simulink model "PC1_DynamicModel"  (R2024b)
settings: Solver=ode45  StartTime=0.0  StopTime=1000  RelTol=1e-3
settings Model: Creator=dereckbouchard  LastModifiedBy=dereckbouchard

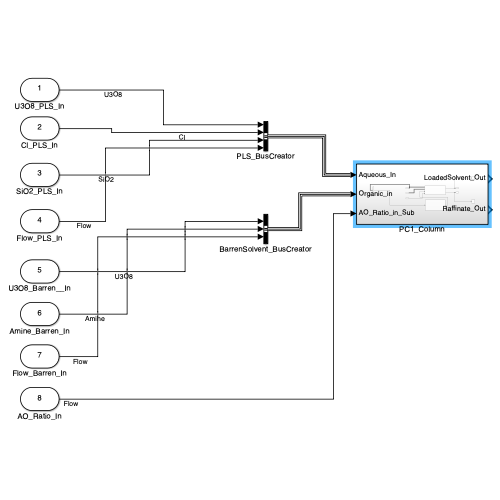
[thumbnail: Simulink's stored preview of the top-level diagram]
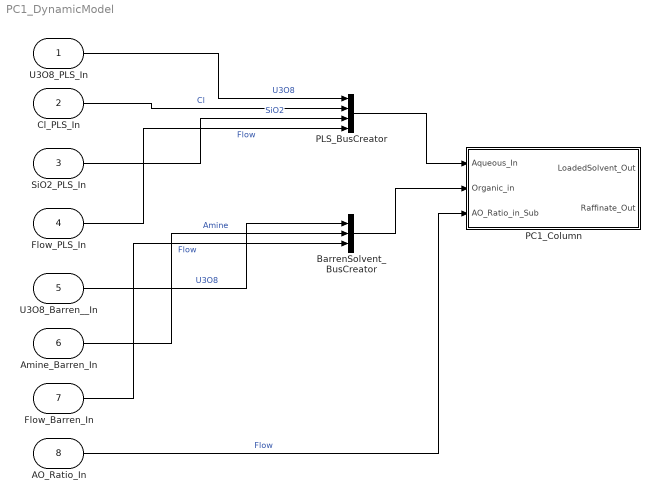
== system PC1_DynamicModel ==
  U3O8_PLS_In : Inport  OutDataTypeStr=double  PortDimensions=[1 1]  SampleTime=0
  Cl_PLS_In : Inport  Port=2  OutDataTypeStr=double  PortDimensions=[1 1]  SampleTime=0
  SiO2_PLS_In : Inport  Port=3  OutDataTypeStr=double  PortDimensions=[1 1]  SampleTime=0
  Flow_PLS_In : Inport  Port=4  OutDataTypeStr=double  PortDimensions=[1 1]  SampleTime=0
  U3O8_Barren__In : Inport  Port=5  OutDataTypeStr=double  PortDimensions=[1 1]  SampleTime=0
  Amine_Barren_In : Inport  Port=6  OutDataTypeStr=double  PortDimensions=[1 1]  SampleTime=0
  Flow_Barren_In : Inport  Port=7  OutDataTypeStr=double  PortDimensions=[1 1]  SampleTime=0
  AO_Ratio_In : Inport  Port=8  OutDataTypeStr=double  PortDimensions=[1 1]  SampleTime=0
  BarrenSolvent_BusCreator : BusCreator  Inputs=3  OutDataTypeStr=Bus: BarrenSolvent_Bus
  PC1_Column : Subsystem
  PLS_BusCreator : BusCreator  Inputs=4  OutDataTypeStr=Bus: PLS_Bus
      settings: InheritFromInputs=off
  wires:
  U3O8_PLS_In/1 -> PLS_BusCreator/1  "U3O8"
  Cl_PLS_In/1 -> PLS_BusCreator/2  "Cl"
  SiO2_PLS_In/1 -> PLS_BusCreator/3  "SiO2"
  Flow_PLS_In/1 -> PLS_BusCreator/4  "Flow"
  U3O8_Barren__In/1 -> BarrenSolvent_BusCreator/1  "U3O8"
  Amine_Barren_In/1 -> BarrenSolvent_BusCreator/2  "Amine"
  Flow_Barren_In/1 -> BarrenSolvent_BusCreator/3  "Flow"
  PLS_BusCreator/1 -> PC1_Column/1(Aqueous_In)
  BarrenSolvent_BusCreator/1 -> PC1_Column/2(Organic_in)
  AO_Ratio_In/1 -> PC1_Column/3(AO_Ratio_in_Sub)  "Flow"

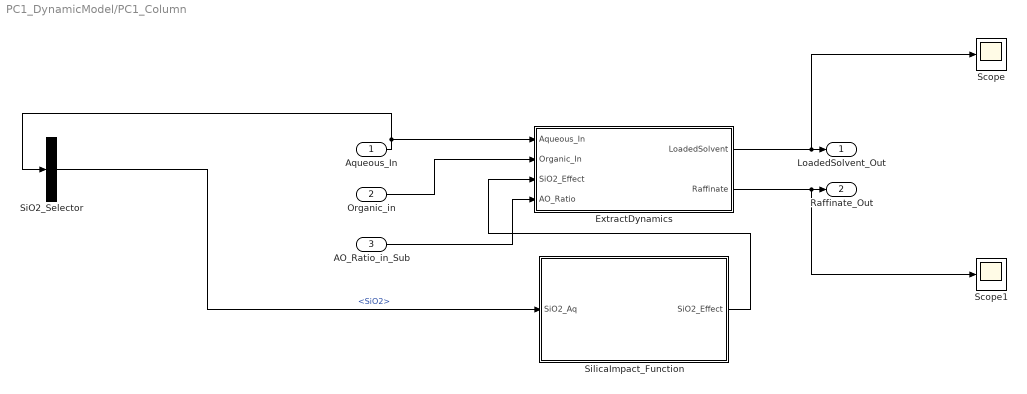
== system PC1_DynamicModel/PC1_Column ==
  Aqueous_In : Inport
  Organic_in : Inport  Port=2
  AO_Ratio_in_Sub : Inport  Port=3
  ExtractDynamics : MATLAB Function  TreatAsAtomicUnit=on
  Scope : Scope
  Scope1 : Scope
  SiO2_Selector : BusSelector  OutputSignals=SiO2
  SilicaImpact_Function : MATLAB Function  TreatAsAtomicUnit=on
  LoadedSolvent_Out : Outport  OutDataTypeStr=double  PortDimensions=[1 3]  SampleTime=0
  Raffinate_Out : Outport  Port=2  OutDataTypeStr=double  PortDimensions=[1 4]  SampleTime=0
  wires:
  Aqueous_In/1 -> SiO2_Selector/1, ExtractDynamics/1(Aqueous_In)
  Organic_in/1 -> ExtractDynamics/2(Organic_In)
  ExtractDynamics/1(LoadedSolvent) -> Scope/1, LoadedSolvent_Out/1
  ExtractDynamics/2(Raffinate) -> Scope1/1, Raffinate_Out/1
  SiO2_Selector/1 -> SilicaImpact_Function/1(SiO2_Aq)  "<SiO2>"
  SilicaImpact_Function/1(SiO2_Effect) -> ExtractDynamics/3(SiO2_Effect)
  AO_Ratio_in_Sub/1 -> ExtractDynamics/4(AO_Ratio)

== matlab function PC1_DynamicModel/PC1_Column/SilicaImpact_Function ==
  data: SiO2_Aq input; SiO2_Effect output
function SiO2_Effect = SilicaImpact(SiO2_Aq)
    % Simplified: Reduces extraction efficiency if SiO2 > 0.4 g/L
    if SiO2_Aq > 0.4
        SiO2_Effect = 0.9; % 10% reduction in efficiency (e.g., entrainment)
    else
        SiO2_Effect = 1.0; % No effect
    end
end

== matlab function PC1_DynamicModel/PC1_Column/ExtractDynamics ==
  data: Aqueous_In input; LoadedSolvent output; Organic_In input; Raffinate output; SiO2_Effect input; AO_Ratio input
function [LoadedSolvent, Raffinate] = ExtractDynamics(Aqueous_In, Organic_In, SiO2_Effect, AO_Ratio)
    % Inputs: Aqueous_In (bus with U3O8, Cl, SiO2, Flow), Organic_In (bus with U3O8, Amine, Flow), SiO2_Effect, AO_Ratio
    % Constants from plant data
    Amine_Conc = 0.06; % 6% amine concentration
    
    % Extract concentrations and flows from buses
    U3O8_Aq = Aqueous_In.U3O8; % mg/L
    Cl_Aq = Aqueous_In.Cl; % mg/L
    SiO2_Aq = Aqueous_In.SiO2; % g/L
    Flow_Aq = Aqueous_In.Flow; % m³/h
    U3O8_Org = Organic_In.U3O8; % mg/L
    Amine_Frac = Organic_In.Amine; % fraction (0.06)
    Flow_Org = Organic_In.Flow; % m³/h
    
    % Uranium extraction reaction (simplified), adjusted for silica and A/O ratio
    % [(R3NH+)_2SO4^2-] + UO2(SO4)2^2- -> [(R3NH+)_2UO2(SO4)2] + SO4^2-
    Max_U3O8_Org = 2500; % Target loaded solvent U3O8 (midpoint of 2100–3150 mg/L)
    U3O8_Extracted = min(U3O8_Aq * (Flow_Aq / (Flow_Aq + Flow_Org * AO_Ratio)), Amine_Frac * 1000 * 1000) * SiO2_Effect;
    
    % Chloride competition reaction
    % [(R3NH+)_2SO4^2-] + Cl- -> (R3NH+Cl-) + SO4^2-
    Cl_Competed = min(Cl_Aq * (Flow_Aq / (Flow_Aq + Flow_Org * AO_Ratio)), Amine_Frac * 1000 * 35.5); % Chloride binding (35.5 g/mol for Cl)
    
    % Update concentrations
    U3O8_Org_New = U3O8_Org + U3O8_Extracted;
    U3O8_Aq_New = U3O8_Aq - U3O8_Extracted;
    Cl_Aq_New = Cl_Aq - Cl_Competed; % Reduced by competition
    SiO2_Aq_New = SiO2_Aq; % Simplified, no extraction but affects entrainment
    
    % Cap at maximum loading (e.g., McCabe-Thiele)
    U3O8_Org_New = min(U3O8_Org_New, Max_U3O8_Org);
    
    % Outputs: Loaded solvent [U3O8, Amine, Flow], Raffinate [U3O8, Cl, SiO2, Flow]
    LoadedSolvent = [U3O8_Org_New, Amine_Frac, Flow_Org];
    Raffinate = [U3O8_Aq_New, Cl_Aq_New, SiO2_Aq_New, Flow_Aq];
end
